simulink model "UoA_1"  (R2014b)
settings: Solver=ode1  StartTime=0.0  StopTime=10000  FixedStep=0.01  RelTol=1e-3
libraries: UoA_3D_LRd_2008 x100
settings Model: SimulationMode=rapid-accelerator  Creator=eyip002-admin  LastModifiedBy=nall426
settings DataIOCC: LimitDataPoints=off  SignalLogging=off  DSMLogging=off  VisualizeSimOutput=off
settings HardwareCC: ProdHWDeviceType=ASIC/FPGA->ASIC/FPGA  TargetBitPerLong=64  TargetBitPerPointer=64  TargetIntDivRoundTo=Zero  TargetEndianess=LittleEndian  TargetWordSize=64  TargetHWDeviceType=Intel->x86-64  ProdEqTarget=off
settings GRTTargetCC: MatFileLogging=off

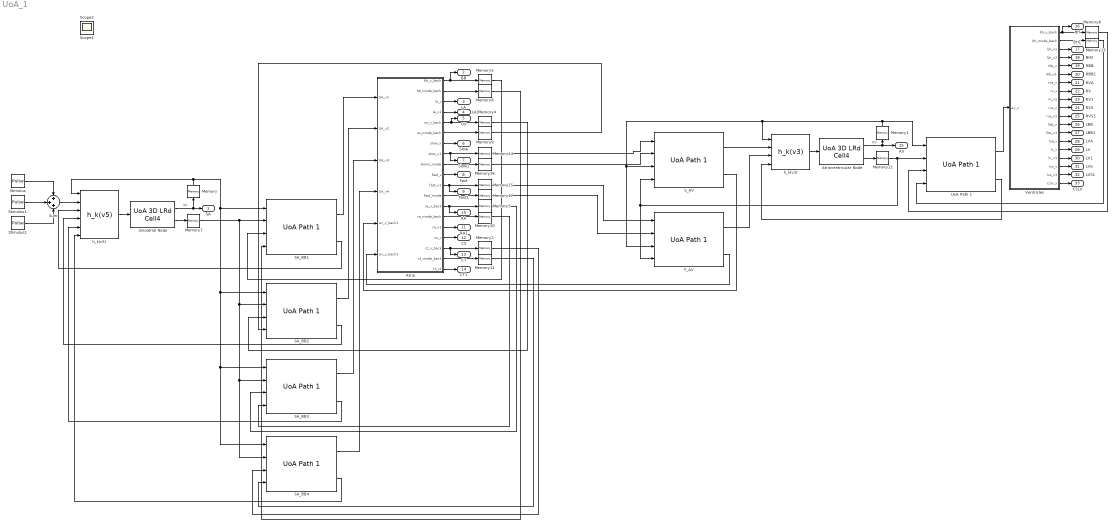
== system UoA_1 ==
  Atria : Subsystem
  Atrioventricular Node : UoA_3D_LRd_2008/UoA 3D LRd Cell4  V_T=44.5  V_R=30  V_O_max=131.1  alpha0_x=-0.0087  alpha1_x=-0.0236  alpha2_x=-0.0069  alpha3_x=-0.0332  alpha0_y=-0.1909  alpha1_y=-0.0455  alpha2_y=0.0759  alpha3_y=0.0200  alpha0_z=-0.1904  alpha1_z=-0.0129  alpha2_z=6.8265  alpha3_z=0.0020  v_n_R_max=0.04  i_st_gx=0.7772  i_st_gy=0.0589  i_st_gz=0.2766
  F_AV : UoA_3D_LRd_2008/UoA Path 1  cell1_conduction_time=10  cell2_conduction_time=10  cell1_charge_time=10  cell2_charge_time=10
  Memory{,1..17} (18 alike) : Memory
  SA_BB{1..4} (4 alike) : UoA_3D_LRd_2008/UoA Path 1  cell1_conduction_time=20  cell2_conduction_time=20  cell1_charge_time=10  cell2_charge_time=10
  S_AV : UoA_3D_LRd_2008/UoA Path 1  cell1_conduction_time=15  cell2_conduction_time=15  cell1_charge_time=10  cell2_charge_time=10
  Sinoatrial Node : UoA_3D_LRd_2008/UoA 3D LRd Cell4  V_T=44.5  V_R=30  V_O_max=131.1  alpha0_x=-0.0087  alpha1_x=-0.0236  alpha2_x=-0.0069  alpha3_x=-0.0332  alpha0_y=-0.1909  alpha1_y=-0.0455  alpha2_y=0.0759  alpha3_y=0.0200  alpha0_z=-0.1904  alpha1_z=-0.0129  alpha2_z=6.8265  alpha3_z=0.0020  v_n_R_max=0.04  i_st_gx=0.7772  i_st_gy=0.0589  i_st_gz=0.2766
  Stimulus : DiscretePulseGenerator  PulseType=Time based  Amplitude=131.1*2  Period=1000  PulseWidth=1.5  PhaseDelay=10
  Stimulus1 : DiscretePulseGenerator  PulseType=Time based  Amplitude=131.1*2  Period=1000  PulseWidth=1.5  PhaseDelay=415
  Stimulus2 : DiscretePulseGenerator  PulseType=Time based  Amplitude=131.1*2  Period=1000  PulseWidth=1.5  PhaseDelay=815
  Sum : Sum  Inputs=+++
  UoA Path 1 : UoA_3D_LRd_2008/UoA Path 1  cell1_conduction_time=30  cell2_conduction_time=30  cell1_charge_time=10  cell2_charge_time=10
  Ventricles : Subsystem
  h_k(v3) : UoA_3D_LRd_2008/h_k(v3)  A_m=10*10  C_m=1/(10*10)  G_1=10*10  G_2=10*10  G_3=10*10  s_1=1/10  s_2=1/10  s_3=1/10  d_1=8  d_2=8  d_3=10
  h_k(v5) : UoA_3D_LRd_2008/h_k(v5)  A_m=10*10  C_m=1/(10*10)  G_1=10*10  G_2=10*10  G_3=10*10  G_4=10*10  G_5=10*10  s_1=1/10  s_2=1/10  s_3=1/10  s_4=1/10  s_5=1/10  d_1=1  d_2=10  d_3=10  d_4=10  d_5=10
  SA : Outport
  BB : Outport  Port=2
  LA : Outport  Port=3
  LA1 : Outport  Port=4
  OS : Outport  Port=5
  Slow : Outport  Port=6
  Slow1 : Outport  Port=7
  Fast : Outport  Port=8
  Fast1 : Outport  Port=9
  RA : Outport  Port=10
  RA1 : Outport  Port=11
  CS : Outport  Port=12
  CT : Outport  Port=13
  CT1 : Outport  Port=14
  AV : Outport  Port=15
  BH : Outport  Port=16
  BH1 : Outport  Port=17
  BH2 : Outport  Port=18
  RBB : Outport  Port=19
  RBB1 : Outport  Port=20
  RVA : Outport  Port=21
  RV : Outport  Port=22
  RV1 : Outport  Port=23
  RVS : Outport  Port=24
  RVS1 : Outport  Port=25
  LBB : Outport  Port=26
  LBB1 : Outport  Port=27
  LVA : Outport  Port=28
  LV : Outport  Port=29
  LV1 : Outport  Port=30
  LVS : Outport  Port=31
  LVS1 : Outport  Port=32
  CSLV : Outport  Port=33
  Scope1 : Scope  NumInputPorts=5
      settings: TimeRange=1000  YMin=-1~-5~-5~-5~-5  YMax=150~150~150~150~150
  Scope2 : Scope  NumInputPorts=12
      settings: TimeRange=1000  YMin=0~-1~-1~-1~-1~-1~-1~-1~-1~-1~-1~-1  YMax=1~1~1~1~1~1~1~1~1~1~1~1  SaveName=ScopeData2
  wires:
  Sinoatrial Node/1 -> SA/1, Memory/1  "SA"
  h_k(v5)/1 -> Sinoatrial Node/1
  Memory/1 -> h_k(v5)/1, SA_BB1/1, SA_BB2/1, SA_BB3/1, SA_BB4/1
  Atrioventricular Node/1 -> AV/1, Memory1/1  "AV"
  Atria/8(slow_v1) -> Slow1/1, Memory14/1
  h_k(v3)/1 -> Atrioventricular Node/1
  Atria/11(fast_v1) -> Fast1/1, Memory15/1
  Ventricles/7(rva_v) -> RVA/1
  Atria/17(ct_v_back) -> CT/1, Memory2/1
  Atria/13(ra_v_back) -> RA/1, Memory3/1
  Atria/5(os_v_back) -> OS/1, Memory4/1
  Atria/1(bb_v_back) -> BB/1, Memory5/1
  Ventricles/1(bh_v_back) -> Memory6/1, BH/1
  Memory2/1 -> SA_BB4/3
  Memory3/1 -> SA_BB3/3
  Memory4/1 -> SA_BB2/3
  Memory5/1 -> SA_BB1/3
  Memory6/1 -> UoA Path 1/3
  Sinoatrial Node/2 -> Memory7/1
  SA_BB1/1 -> Atria/1(SA_v1)
  Atria/2(bb_mode_back) -> Memory8/1
  Memory8/1 -> SA_BB1/4
  SA_BB1/2 -> h_k(v5)/3
  Atria/6(os_mode_back) -> Memory9/1
  Memory9/1 -> SA_BB2/4
  SA_BB2/2 -> h_k(v5)/4
  SA_BB2/1 -> Atria/2(SA_v2)
  Atria/14(ra_mode_back) -> Memory10/1
  Memory10/1 -> SA_BB3/4
  SA_BB3/1 -> Atria/3(SA_v3)
  SA_BB3/2 -> h_k(v5)/5
  Memory7/1 -> SA_BB3/2, SA_BB4/2, SA_BB2/2, SA_BB1/2
  Atria/18(ct_mode_back) -> Memory11/1
  Memory11/1 -> SA_BB4/4
  SA_BB4/1 -> Atria/4(SA_v4)
  SA_BB4/2 -> h_k(v5)/6
  Memory1/1 -> UoA Path 1/1, h_k(v3)/1, F_AV/3, S_AV/3
  Atrioventricular Node/2 -> Memory12/1
  Memory12/1 -> S_AV/4, F_AV/4, UoA Path 1/2
  UoA Path 1/1 -> Ventricles/1(av_v)
  Ventricles/2(bh_mode_back) -> Memory13/1
  Memory13/1 -> UoA Path 1/4
  UoA Path 1/2 -> h_k(v3)/4
  Memory14/1 -> S_AV/1
  Memory15/1 -> F_AV/1
  Atria/9(slow1_mode) -> Memory16/1
  Atria/12(fast_mode) -> Memory17/1
  Memory16/1 -> S_AV/2
  S_AV/1 -> h_k(v3)/2
  S_AV/2 -> Atria/5(av_v_back1)
  Memory17/1 -> F_AV/2
  F_AV/1 -> h_k(v3)/3
  F_AV/2 -> Atria/6(av_v_back2)
  Atria/4(la_v1) -> LA1/1
  Atria/3(la_v) -> LA/1
  Atria/7(slow_v) -> Slow/1
  Atria/10(fast_v) -> Fast/1
  Atria/15(ra_v1) -> RA1/1
  Atria/16(cs_v) -> CS/1
  Atria/19(ct_v1) -> CT1/1
  Ventricles/3(bh_v1) -> BH1/1
  Ventricles/4(bh_v2) -> BH2/1
  Ventricles/5(rbb_v) -> RBB/1
  Ventricles/6(rbb_v1) -> RBB1/1
  Ventricles/8(rv_v) -> RV/1
  Ventricles/9(rv_v1) -> RV1/1
  Ventricles/10(rvs_v) -> RVS/1
  Ventricles/11(rvs_v1) -> RVS1/1
  Ventricles/12(lbb_v) -> LBB/1
  Ventricles/13(lbb_v1) -> LBB1/1
  Ventricles/14(lva_v) -> LVA/1
  Ventricles/15(lv_v) -> LV/1
  Ventricles/16(lv_v1) -> LV1/1
  Ventricles/17(lvs_v) -> LVS/1
  Ventricles/18(lvs_v1) -> LVS1/1
  Ventricles/19(cslv_v) -> CSLV/1
  Sum/1 -> h_k(v5)/2
  Stimulus/1 -> Sum/1
  Stimulus1/1 -> Sum/2
  Stimulus2/1 -> Sum/3

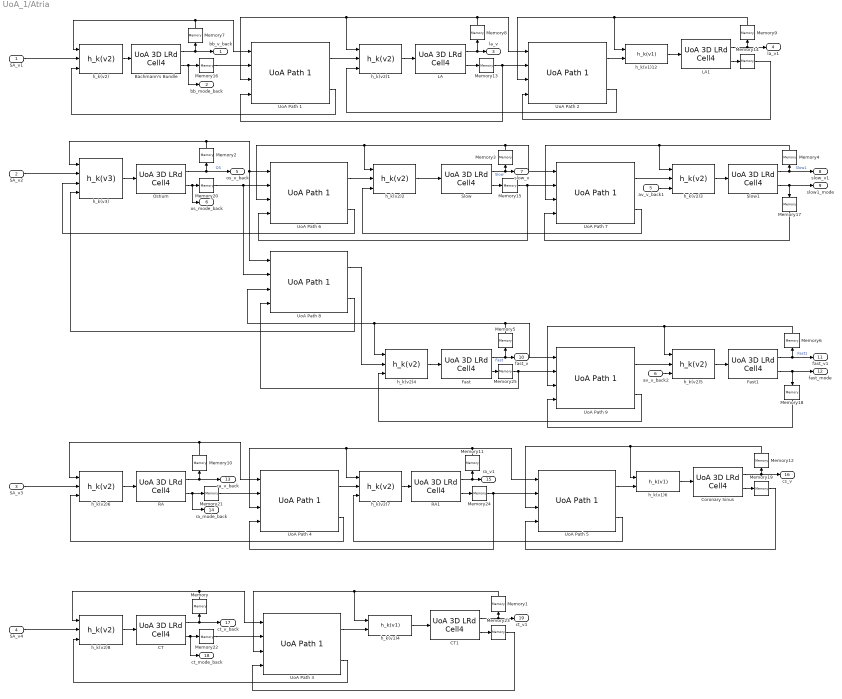
== system UoA_1/Atria ==
  SA_v1 : Inport
  SA_v2 : Inport  Port=2
  SA_v3 : Inport  Port=3
  SA_v4 : Inport  Port=4
  av_v_back1 : Inport  Port=5
  av_v_back2 : Inport  Port=6
  Bachmann's Bundle : UoA_3D_LRd_2008/UoA 3D LRd Cell4  V_T=44.5  V_R=30  V_O_max=131.1  alpha0_x=-0.0087  alpha1_x=-0.0236  alpha2_x=-0.0069  alpha3_x=-0.0332  alpha0_y=-0.1909  alpha1_y=-0.0455  alpha2_y=0.0759  alpha3_y=0.0200  alpha0_z=-0.1904  alpha1_z=-0.0129  alpha2_z=6.8265  alpha3_z=0.0020  v_n_R_max=0.04  i_st_gx=0.7772  i_st_gy=0.0589  i_st_gz=0.2766
  CT : UoA_3D_LRd_2008/UoA 3D LRd Cell4  V_T=44.5  V_R=30  V_O_max=131.1  alpha0_x=-0.0087  alpha1_x=-0.0236  alpha2_x=-0.0069  alpha3_x=-0.0332  alpha0_y=-0.1909  alpha1_y=-0.0455  alpha2_y=0.0759  alpha3_y=0.0200  alpha0_z=-0.1904  alpha1_z=-0.0129  alpha2_z=6.8265  alpha3_z=0.0020  v_n_R_max=0.04  i_st_gx=0.7772  i_st_gy=0.0589  i_st_gz=0.2766
  CT1 : UoA_3D_LRd_2008/UoA 3D LRd Cell4  V_T=44.5  V_R=30  V_O_max=131.1  alpha0_x=-0.0087  alpha1_x=-0.0236  alpha2_x=-0.0069  alpha3_x=-0.0332  alpha0_y=-0.1909  alpha1_y=-0.0455  alpha2_y=0.0759  alpha3_y=0.0200  alpha0_z=-0.1904  alpha1_z=-0.0129  alpha2_z=6.8265  alpha3_z=0.0020  v_n_R_max=0.04  i_st_gx=0.7772  i_st_gy=0.0589  i_st_gz=0.2766
  Coronary Sinus : UoA_3D_LRd_2008/UoA 3D LRd Cell4  V_T=44.5  V_R=30  V_O_max=131.1  alpha0_x=-0.0087  alpha1_x=-0.0236  alpha2_x=-0.0069  alpha3_x=-0.0332  alpha0_y=-0.1909  alpha1_y=-0.0455  alpha2_y=0.0759  alpha3_y=0.0200  alpha0_z=-0.1904  alpha1_z=-0.0129  alpha2_z=6.8265  alpha3_z=0.0020  v_n_R_max=0.04  i_st_gx=0.7772  i_st_gy=0.0589  i_st_gz=0.2766
  Fast : UoA_3D_LRd_2008/UoA 3D LRd Cell4  V_T=44.5  V_R=30  V_O_max=131.1  alpha0_x=-0.0087  alpha1_x=-0.0236  alpha2_x=-0.0069  alpha3_x=-0.0332  alpha0_y=-0.1909  alpha1_y=-0.0455  alpha2_y=0.0759  alpha3_y=0.0180  alpha0_z=-0.1904  alpha1_z=-0.0129  alpha2_z=6.8265  alpha3_z=0.0020  v_n_R_max=0.04  i_st_gx=0.7772  i_st_gy=0.0589  i_st_gz=0.2766
  Fast1 : UoA_3D_LRd_2008/UoA 3D LRd Cell4  V_T=44.5  V_R=30  V_O_max=131.1  alpha0_x=-0.0087  alpha1_x=-0.0236  alpha2_x=-0.0069  alpha3_x=-0.0332  alpha0_y=-0.1909  alpha1_y=-0.0455  alpha2_y=0.0759  alpha3_y=0.0180  alpha0_z=-0.1904  alpha1_z=-0.0129  alpha2_z=6.8265  alpha3_z=0.0020  v_n_R_max=0.04  i_st_gx=0.7772  i_st_gy=0.0589  i_st_gz=0.2766
  LA : UoA_3D_LRd_2008/UoA 3D LRd Cell4  V_T=44.5  V_R=30  V_O_max=131.1  alpha0_x=-0.0087  alpha1_x=-0.0236  alpha2_x=-0.0069  alpha3_x=-0.0332  alpha0_y=-0.1909  alpha1_y=-0.0455  alpha2_y=0.0759  alpha3_y=0.0200  alpha0_z=-0.1904  alpha1_z=-0.0129  alpha2_z=6.8265  alpha3_z=0.0020  v_n_R_max=0.04  i_st_gx=0.7772  i_st_gy=0.0589  i_st_gz=0.2766
  LA1 : UoA_3D_LRd_2008/UoA 3D LRd Cell4  V_T=44.5  V_R=30  V_O_max=131.1  alpha0_x=-0.0087  alpha1_x=-0.0236  alpha2_x=-0.0069  alpha3_x=-0.0332  alpha0_y=-0.1909  alpha1_y=-0.0455  alpha2_y=0.0759  alpha3_y=0.0200  alpha0_z=-0.1904  alpha1_z=-0.0129  alpha2_z=6.8265  alpha3_z=0.0020  v_n_R_max=0.04  i_st_gx=0.7772  i_st_gy=0.0589  i_st_gz=0.2766
  Memory{,1..25} (26 alike) : Memory
  Ostium : UoA_3D_LRd_2008/UoA 3D LRd Cell4  V_T=44.5  V_R=30  V_O_max=131.1  alpha0_x=-0.0087  alpha1_x=-0.0236  alpha2_x=-0.0069  alpha3_x=-0.0332  alpha0_y=-0.1909  alpha1_y=-0.0455  alpha2_y=0.0759  alpha3_y=0.0200  alpha0_z=-0.1904  alpha1_z=-0.0129  alpha2_z=6.8265  alpha3_z=0.0020  v_n_R_max=0.04  i_st_gx=0.7772  i_st_gy=0.0589  i_st_gz=0.2766
  RA : UoA_3D_LRd_2008/UoA 3D LRd Cell4  V_T=44.5  V_R=30  V_O_max=131.1  alpha0_x=-0.0087  alpha1_x=-0.0236  alpha2_x=-0.0069  alpha3_x=-0.0332  alpha0_y=-0.1909  alpha1_y=-0.0455  alpha2_y=0.0759  alpha3_y=0.0200  alpha0_z=-0.1904  alpha1_z=-0.0129  alpha2_z=6.8265  alpha3_z=0.0020  v_n_R_max=0.04  i_st_gx=0.7772  i_st_gy=0.0589  i_st_gz=0.2766
  RA1 : UoA_3D_LRd_2008/UoA 3D LRd Cell4  V_T=44.5  V_R=30  V_O_max=131.1  alpha0_x=-0.0087  alpha1_x=-0.0236  alpha2_x=-0.0069  alpha3_x=-0.0332  alpha0_y=-0.1909  alpha1_y=-0.0455  alpha2_y=0.0759  alpha3_y=0.0200  alpha0_z=-0.1904  alpha1_z=-0.0129  alpha2_z=6.8265  alpha3_z=0.0020  v_n_R_max=0.04  i_st_gx=0.7772  i_st_gy=0.0589  i_st_gz=0.2766
  Slow : UoA_3D_LRd_2008/UoA 3D LRd Cell4  V_T=44.5  V_R=30  V_O_max=131.1  alpha0_x=-0.0087  alpha1_x=-0.0236  alpha2_x=-0.0069  alpha3_x=-0.0332  alpha0_y=-0.1909  alpha1_y=-0.0455  alpha2_y=0.0759  alpha3_y=0.0200  alpha0_z=-0.1904  alpha1_z=-0.0129  alpha2_z=6.8265  alpha3_z=0.0020  v_n_R_max=0.04  i_st_gx=0.7772  i_st_gy=0.0589  i_st_gz=0.2766
  Slow1 : UoA_3D_LRd_2008/UoA 3D LRd Cell4  V_T=44.5  V_R=30  V_O_max=131.1  alpha0_x=-0.0087  alpha1_x=-0.0236  alpha2_x=-0.0069  alpha3_x=-0.0332  alpha0_y=-0.1909  alpha1_y=-0.0455  alpha2_y=0.0759  alpha3_y=0.0200  alpha0_z=-0.1904  alpha1_z=-0.0129  alpha2_z=6.8265  alpha3_z=0.0020  v_n_R_max=0.04  i_st_gx=0.7772  i_st_gy=0.0589  i_st_gz=0.2766
  UoA Path 1 : UoA_3D_LRd_2008/UoA Path 1  cell1_conduction_time=30  cell2_conduction_time=30  cell1_charge_time=10  cell2_charge_time=10
  UoA Path 2 : UoA_3D_LRd_2008/UoA Path 1  cell1_conduction_time=40  cell2_conduction_time=40  cell1_charge_time=10  cell2_charge_time=10
  UoA Path {3..5,8..9} (5 alike) : UoA_3D_LRd_2008/UoA Path 1  cell1_conduction_time=20  cell2_conduction_time=20  cell1_charge_time=10  cell2_charge_time=10
  UoA Path 6 : UoA_3D_LRd_2008/UoA Path 1  cell1_conduction_time=30  cell2_conduction_time=30  cell1_charge_time=10  cell2_charge_time=10
  UoA Path 7 : UoA_3D_LRd_2008/UoA Path 1  cell1_conduction_time=30  cell2_conduction_time=30  cell1_charge_time=10  cell2_charge_time=10
  h_k(v1)12 : UoA_3D_LRd_2008/h_k(v1)  A_m=10*10  C_m=1/(10*10)  G_1=10*10  s_1=1/10  d_1=10
  h_k(v1)4 : UoA_3D_LRd_2008/h_k(v1)  A_m=10*10  C_m=1/(10*10)  G_1=10*10  s_1=1/10  d_1=10
  h_k(v1)6 : UoA_3D_LRd_2008/h_k(v1)  A_m=10*10  C_m=1/(10*10)  G_1=10*10  s_1=1/10  d_1=10
  h_k(v2){,1..8} (9 alike) : UoA_3D_LRd_2008/h_k(v2)  A_m=10*10  C_m=1/(10*10)  G_1=10*10  G_2=10*10  s_1=1/10  s_2=1/10  d_1=10  d_2=10
  h_k(v3) : UoA_3D_LRd_2008/h_k(v3)  A_m=10*10  C_m=1/(10*10)  G_1=10*10  G_2=10*10  G_3=10*10  s_1=1/10  s_2=1/10  s_3=1/10  d_1=1  d_2=10  d_3=10
  bb_v_back : Outport
  bb_mode_back : Outport  Port=2
  la_v : Outport  Port=3
  la_v1 : Outport  Port=4
  os_v_back : Outport  Port=5
  os_mode_back : Outport  Port=6
  slow_v : Outport  Port=7
  slow_v1 : Outport  Port=8
  slow1_mode : Outport  Port=9
  fast_v : Outport  Port=10
  fast_v1 : Outport  Port=11
  fast_mode : Outport  Port=12
  ra_v_back : Outport  Port=13
  ra_mode_back : Outport  Port=14
  ra_v1 : Outport  Port=15
  cs_v : Outport  Port=16
  ct_v_back : Outport  Port=17
  ct_mode_back : Outport  Port=18
  ct_v1 : Outport  Port=19
  wires:
  CT/1 -> Memory/1, ct_v_back/1
  CT1/1 -> ct_v1/1, Memory1/1
  h_k(v2)8/1 -> CT/1
  Memory/1 -> h_k(v2)8/1, UoA Path 3/1
  h_k(v1)4/1 -> CT1/1
  Memory1/1 -> UoA Path 3/3, h_k(v1)4/1
  h_k(v3)/1 -> Ostium/1
  Memory2/1 -> h_k(v3)/1, UoA Path 8/1, UoA Path 6/1
  SA_v1/1 -> h_k(v2)/2
  h_k(v2)2/1 -> Slow/1
  Memory3/1 -> UoA Path 6/3, h_k(v2)2/1, UoA Path 7/1
  h_k(v2)3/1 -> Slow1/1
  Memory4/1 -> h_k(v2)3/1, UoA Path 7/3
  Slow/1 -> slow_v/1, Memory3/1  "Slow"
  h_k(v2)4/1 -> Fast/1
  Ostium/1 -> Memory2/1, os_v_back/1  "OS"
  h_k(v2)5/1 -> Fast1/1
  Memory6/1 -> h_k(v2)5/1, UoA Path 9/3
  Fast/1 -> fast_v/1, Memory5/1  "Fast"
  Slow1/1 -> slow_v1/1, Memory4/1  "Slow1"
  Fast1/1 -> fast_v1/1, Memory6/1  "Fast1"
  h_k(v2)/1 -> Bachmann's Bundle/1
  Memory7/1 -> UoA Path 1/1, h_k(v2)/1
  h_k(v2)1/1 -> LA/1
  Memory8/1 -> UoA Path 2/1, h_k(v2)1/1, UoA Path 1/3
  h_k(v1)12/1 -> LA1/1
  Memory9/1 -> h_k(v1)12/1, UoA Path 2/3
  LA/1 -> la_v/1, Memory8/1
  Bachmann's Bundle/1 -> bb_v_back/1, Memory7/1
  LA1/1 -> la_v1/1, Memory9/1
  h_k(v2)6/1 -> RA/1
  Memory10/1 -> h_k(v2)6/1, UoA Path 4/1
  h_k(v2)7/1 -> RA1/1
  Memory11/1 -> h_k(v2)7/1, UoA Path 4/3, UoA Path 5/1
  h_k(v1)6/1 -> Coronary Sinus/1
  Memory12/1 -> h_k(v1)6/1, UoA Path 5/3
  RA1/1 -> ra_v1/1, Memory11/1
  RA/1 -> ra_v_back/1, Memory10/1
  Coronary Sinus/1 -> cs_v/1, Memory12/1
  av_v_back1/1 -> h_k(v2)3/3
  Memory14/1 -> UoA Path 2/4
  UoA Path 6/2 -> h_k(v3)/3
  Memory5/1 -> h_k(v2)4/1, UoA Path 8/3, UoA Path 9/1
  UoA Path 7/2 -> h_k(v2)2/3
  LA1/2 -> Memory14/1
  CT1/2 -> Memory23/1
  Slow1/2 -> Memory17/1, slow1_mode/1
  Fast1/2 -> Memory18/1, fast_mode/1
  Ostium/2 -> Memory20/1, os_mode_back/1
  SA_v2/1 -> h_k(v3)/2
  SA_v3/1 -> h_k(v2)6/2
  SA_v4/1 -> h_k(v2)8/2
  av_v_back2/1 -> h_k(v2)5/3
  LA/2 -> Memory13/1
  Memory13/1 -> UoA Path 1/4, UoA Path 2/2
  UoA Path 1/1 -> h_k(v2)1/2
  UoA Path 1/2 -> h_k(v2)/3
  UoA Path 2/2 -> h_k(v2)1/3
  UoA Path 2/1 -> h_k(v1)12/2
  Bachmann's Bundle/2 -> Memory16/1, bb_mode_back/1
  UoA Path 3/1 -> h_k(v1)4/2
  CT/2 -> ct_mode_back/1, Memory22/1
  Memory23/1 -> UoA Path 3/4
  UoA Path 3/2 -> h_k(v2)8/3
  RA/2 -> ra_mode_back/1, Memory21/1
  UoA Path 4/1 -> h_k(v2)7/2
  RA1/2 -> Memory24/1
  Memory24/1 -> UoA Path 5/2, UoA Path 4/4
  UoA Path 4/2 -> h_k(v2)6/3
  UoA Path 5/1 -> h_k(v1)6/2
  UoA Path 5/2 -> h_k(v2)7/3
  Coronary Sinus/2 -> Memory19/1
  Memory19/1 -> UoA Path 5/4
  Memory21/1 -> UoA Path 4/2
  Memory22/1 -> UoA Path 3/2
  Memory16/1 -> UoA Path 1/2
  Memory20/1 -> UoA Path 8/2, UoA Path 6/2
  UoA Path 6/1 -> h_k(v2)2/2
  Slow/2 -> Memory15/1
  Memory15/1 -> UoA Path 7/2, UoA Path 6/4
  Memory17/1 -> UoA Path 7/4
  UoA Path 7/1 -> h_k(v2)3/2
  UoA Path 8/1 -> h_k(v2)4/2
  UoA Path 8/2 -> h_k(v3)/4
  Fast/2 -> Memory25/1
  Memory25/1 -> UoA Path 9/2, UoA Path 8/4
  UoA Path 9/2 -> h_k(v2)4/3
  UoA Path 9/1 -> h_k(v2)5/2
  Memory18/1 -> UoA Path 9/4

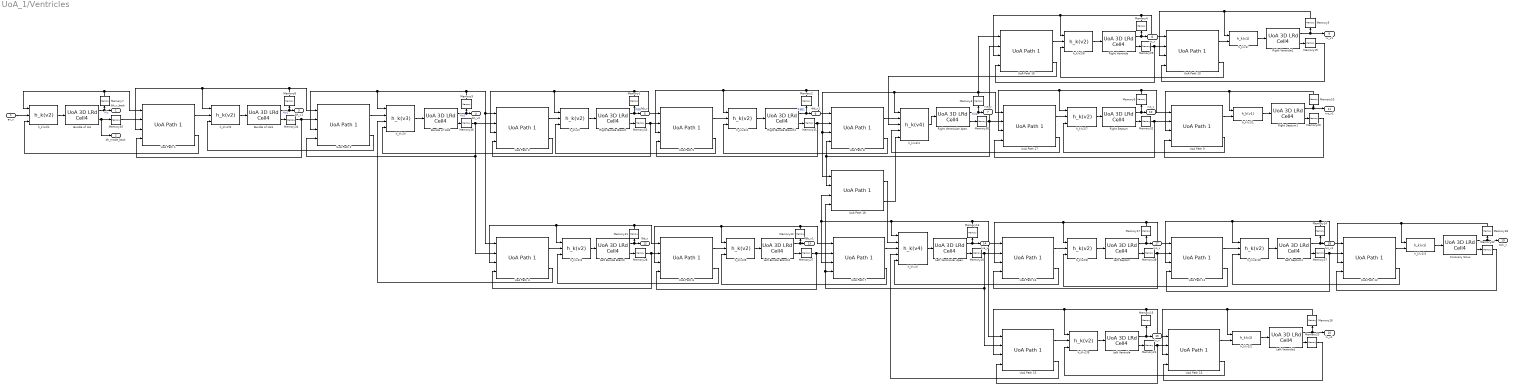
== system UoA_1/Ventricles ==
  av_v : Inport
  Bundle of His : UoA_3D_LRd_2008/UoA 3D LRd Cell4  V_T=44.5  V_R=30  V_O_max=131.1  alpha0_x=-0.0087  alpha1_x=-0.0236  alpha2_x=-0.0069  alpha3_x=-0.0332  alpha0_y=-0.1909  alpha1_y=-0.0455  alpha2_y=0.0759  alpha3_y=0.0110  alpha0_z=-0.1904  alpha1_z=-0.0129  alpha2_z=6.8265  alpha3_z=0.0020  v_n_R_max=0.04  i_st_gx=0.7772  i_st_gy=0.0589  i_st_gz=0.2766
  Bundle of His1 : UoA_3D_LRd_2008/UoA 3D LRd Cell4  V_T=44.5  V_R=30  V_O_max=131.1  alpha0_x=-0.0087  alpha1_x=-0.0236  alpha2_x=-0.0069  alpha3_x=-0.0332  alpha0_y=-0.1909  alpha1_y=-0.0455  alpha2_y=0.0759  alpha3_y=0.0110  alpha0_z=-0.1904  alpha1_z=-0.0129  alpha2_z=6.8265  alpha3_z=0.0020  v_n_R_max=0.04  i_st_gx=0.7772  i_st_gy=0.0589  i_st_gz=0.2766
  Bundle of His2 : UoA_3D_LRd_2008/UoA 3D LRd Cell4  V_T=44.5  V_R=30  V_O_max=131.1  alpha0_x=-0.0087  alpha1_x=-0.0236  alpha2_x=-0.0069  alpha3_x=-0.0332  alpha0_y=-0.1909  alpha1_y=-0.0455  alpha2_y=0.0759  alpha3_y=0.0110  alpha0_z=-0.1904  alpha1_z=-0.0129  alpha2_z=6.8265  alpha3_z=0.0020  v_n_R_max=0.04  i_st_gx=0.7772  i_st_gy=0.0589  i_st_gz=0.2766
  Coronary Sinus : UoA_3D_LRd_2008/UoA 3D LRd Cell4  V_T=44.5  V_R=30  V_O_max=131.1  alpha0_x=-0.0087  alpha1_x=-0.0236  alpha2_x=-0.0069  alpha3_x=-0.0332  alpha0_y=-0.1909  alpha1_y=-0.0455  alpha2_y=0.0759  alpha3_y=0.0110  alpha0_z=-0.1904  alpha1_z=-0.0129  alpha2_z=6.8265  alpha3_z=0.0020  v_n_R_max=0.04  i_st_gx=0.7772  i_st_gy=0.0589  i_st_gz=0.2766
  Left Bundle Branch : UoA_3D_LRd_2008/UoA 3D LRd Cell4  V_T=44.5  V_R=30  V_O_max=131.1  alpha0_x=-0.0087  alpha1_x=-0.0236  alpha2_x=-0.0069  alpha3_x=-0.0332  alpha0_y=-0.1909  alpha1_y=-0.0455  alpha2_y=0.0759  alpha3_y=0.0110  alpha0_z=-0.1904  alpha1_z=-0.0129  alpha2_z=6.8265  alpha3_z=0.0020  v_n_R_max=0.04  i_st_gx=0.7772  i_st_gy=0.0589  i_st_gz=0.2766
  Left Bundle Branch1 : UoA_3D_LRd_2008/UoA 3D LRd Cell4  V_T=44.5  V_R=30  V_O_max=131.1  alpha0_x=-0.0087  alpha1_x=-0.0236  alpha2_x=-0.0069  alpha3_x=-0.0332  alpha0_y=-0.1909  alpha1_y=-0.0455  alpha2_y=0.0759  alpha3_y=0.0110  alpha0_z=-0.1904  alpha1_z=-0.0129  alpha2_z=6.8265  alpha3_z=0.0020  v_n_R_max=0.04  i_st_gx=0.7772  i_st_gy=0.0589  i_st_gz=0.2766
  Left Septum : UoA_3D_LRd_2008/UoA 3D LRd Cell4  V_T=44.5  V_R=30  V_O_max=131.1  alpha0_x=-0.0087  alpha1_x=-0.0236  alpha2_x=-0.0069  alpha3_x=-0.0332  alpha0_y=-0.1909  alpha1_y=-0.0455  alpha2_y=0.0759  alpha3_y=0.0110  alpha0_z=-0.1904  alpha1_z=-0.0129  alpha2_z=6.8265  alpha3_z=0.0020  v_n_R_max=0.04  i_st_gx=0.7772  i_st_gy=0.0589  i_st_gz=0.2766
  Left Septum1 : UoA_3D_LRd_2008/UoA 3D LRd Cell4  V_T=44.5  V_R=30  V_O_max=131.1  alpha0_x=-0.0087  alpha1_x=-0.0236  alpha2_x=-0.0069  alpha3_x=-0.0332  alpha0_y=-0.1909  alpha1_y=-0.0455  alpha2_y=0.0759  alpha3_y=0.0110  alpha0_z=-0.1904  alpha1_z=-0.0129  alpha2_z=6.8265  alpha3_z=0.0020  v_n_R_max=0.04  i_st_gx=0.7772  i_st_gy=0.0589  i_st_gz=0.2766
  Left Ventricle : UoA_3D_LRd_2008/UoA 3D LRd Cell4  V_T=44.5  V_R=30  V_O_max=131.1  alpha0_x=-0.0087  alpha1_x=-0.0236  alpha2_x=-0.0069  alpha3_x=-0.0332  alpha0_y=-0.1909  alpha1_y=-0.0455  alpha2_y=0.0759  alpha3_y=0.0110  alpha0_z=-0.1904  alpha1_z=-0.0129  alpha2_z=6.8265  alpha3_z=0.0020  v_n_R_max=0.04  i_st_gx=0.7772  i_st_gy=0.0589  i_st_gz=0.2766
  Left Ventricle1 : UoA_3D_LRd_2008/UoA 3D LRd Cell4  V_T=44.5  V_R=30  V_O_max=131.1  alpha0_x=-0.0087  alpha1_x=-0.0236  alpha2_x=-0.0069  alpha3_x=-0.0332  alpha0_y=-0.1909  alpha1_y=-0.0455  alpha2_y=0.0759  alpha3_y=0.0110  alpha0_z=-0.1904  alpha1_z=-0.0129  alpha2_z=6.8265  alpha3_z=0.0020  v_n_R_max=0.04  i_st_gx=0.7772  i_st_gy=0.0589  i_st_gz=0.2766
  Left Ventricular Apex : UoA_3D_LRd_2008/UoA 3D LRd Cell4  V_T=44.5  V_R=30  V_O_max=131.1  alpha0_x=-0.0087  alpha1_x=-0.0236  alpha2_x=-0.0069  alpha3_x=-0.0332  alpha0_y=-0.1909  alpha1_y=-0.0455  alpha2_y=0.0759  alpha3_y=0.0110  alpha0_z=-0.1904  alpha1_z=-0.0129  alpha2_z=6.8265  alpha3_z=0.0020  v_n_R_max=0.04  i_st_gx=0.7772  i_st_gy=0.0589  i_st_gz=0.2766
  Memory{1..23,26..38} (36 alike) : Memory
  Right Bundle Branch : UoA_3D_LRd_2008/UoA 3D LRd Cell4  V_T=44.5  V_R=30  V_O_max=131.1  alpha0_x=-0.0087  alpha1_x=-0.0236  alpha2_x=-0.0069  alpha3_x=-0.0332  alpha0_y=-0.1909  alpha1_y=-0.0455  alpha2_y=0.0759  alpha3_y=0.0110  alpha0_z=-0.1904  alpha1_z=-0.0129  alpha2_z=6.8265  alpha3_z=0.0020  v_n_R_max=0.04  i_st_gx=0.7772  i_st_gy=0.0589  i_st_gz=0.2766
  Right Bundle Branch1 : UoA_3D_LRd_2008/UoA 3D LRd Cell4  V_T=44.5  V_R=30  V_O_max=131.1  alpha0_x=-0.0087  alpha1_x=-0.0236  alpha2_x=-0.0069  alpha3_x=-0.0332  alpha0_y=-0.1909  alpha1_y=-0.0455  alpha2_y=0.0759  alpha3_y=0.0110  alpha0_z=-0.1904  alpha1_z=-0.0129  alpha2_z=6.8265  alpha3_z=0.0020  v_n_R_max=0.04  i_st_gx=0.7772  i_st_gy=0.0589  i_st_gz=0.2766
  Right Septum : UoA_3D_LRd_2008/UoA 3D LRd Cell4  V_T=44.5  V_R=30  V_O_max=131.1  alpha0_x=-0.0087  alpha1_x=-0.0236  alpha2_x=-0.0069  alpha3_x=-0.0332  alpha0_y=-0.1909  alpha1_y=-0.0455  alpha2_y=0.0759  alpha3_y=0.0110  alpha0_z=-0.1904  alpha1_z=-0.0129  alpha2_z=6.8265  alpha3_z=0.0020  v_n_R_max=0.04  i_st_gx=0.7772  i_st_gy=0.0589  i_st_gz=0.2766
  Right Septum1 : UoA_3D_LRd_2008/UoA 3D LRd Cell4  V_T=44.5  V_R=30  V_O_max=131.1  alpha0_x=-0.0087  alpha1_x=-0.0236  alpha2_x=-0.0069  alpha3_x=-0.0332  alpha0_y=-0.1909  alpha1_y=-0.0455  alpha2_y=0.0759  alpha3_y=0.0110  alpha0_z=-0.1904  alpha1_z=-0.0129  alpha2_z=6.8265  alpha3_z=0.0020  v_n_R_max=0.04  i_st_gx=0.7772  i_st_gy=0.0589  i_st_gz=0.2766
  Right Ventricle : UoA_3D_LRd_2008/UoA 3D LRd Cell4  V_T=44.5  V_R=30  V_O_max=131.1  alpha0_x=-0.0087  alpha1_x=-0.0236  alpha2_x=-0.0069  alpha3_x=-0.0332  alpha0_y=-0.1909  alpha1_y=-0.0455  alpha2_y=0.0759  alpha3_y=0.0110  alpha0_z=-0.1904  alpha1_z=-0.0129  alpha2_z=6.8265  alpha3_z=0.0020  v_n_R_max=0.04  i_st_gx=0.7772  i_st_gy=0.0589  i_st_gz=0.2766
  Right Ventricle1 : UoA_3D_LRd_2008/UoA 3D LRd Cell4  V_T=44.5  V_R=30  V_O_max=131.1  alpha0_x=-0.0087  alpha1_x=-0.0236  alpha2_x=-0.0069  alpha3_x=-0.0332  alpha0_y=-0.1909  alpha1_y=-0.0455  alpha2_y=0.0759  alpha3_y=0.0110  alpha0_z=-0.1904  alpha1_z=-0.0129  alpha2_z=6.8265  alpha3_z=0.0020  v_n_R_max=0.04  i_st_gx=0.7772  i_st_gy=0.0589  i_st_gz=0.2766
  Right Ventricular Apex : UoA_3D_LRd_2008/UoA 3D LRd Cell4  V_T=44.5  V_R=30  V_O_max=131.1  alpha0_x=-0.0087  alpha1_x=-0.0236  alpha2_x=-0.0069  alpha3_x=-0.0332  alpha0_y=-0.1909  alpha1_y=-0.0455  alpha2_y=0.0759  alpha3_y=0.0110  alpha0_z=-0.1904  alpha1_z=-0.0129  alpha2_z=6.8265  alpha3_z=0.0020  v_n_R_max=0.04  i_st_gx=0.7772  i_st_gy=0.0589  i_st_gz=0.2766
  UoA Path {1..4,9..10,12,15} (8 alike) : UoA_3D_LRd_2008/UoA Path 1  cell1_conduction_time=20  cell2_conduction_time=20  cell1_charge_time=10  cell2_charge_time=10
  UoA Path 11 : UoA_3D_LRd_2008/UoA Path 1  cell1_conduction_time=15  cell2_conduction_time=15  cell1_charge_time=10  cell2_charge_time=10
  UoA Path 13 : UoA_3D_LRd_2008/UoA Path 1  cell1_conduction_time=30  cell2_conduction_time=30  cell1_charge_time=10  cell2_charge_time=10
  UoA Path 14 : UoA_3D_LRd_2008/UoA Path 1  cell1_conduction_time=15  cell2_conduction_time=15  cell1_charge_time=10  cell2_charge_time=10
  UoA Path 16 : UoA_3D_LRd_2008/UoA Path 1  cell1_conduction_time=10  cell2_conduction_time=10  cell1_charge_time=10  cell2_charge_time=10
  UoA Path 17 : UoA_3D_LRd_2008/UoA Path 1  cell1_conduction_time=15  cell2_conduction_time=15  cell1_charge_time=10  cell2_charge_time=10
  UoA Path {5..8,18} (5 alike) : UoA_3D_LRd_2008/UoA Path 1  cell1_conduction_time=5  cell2_conduction_time=5  cell1_charge_time=10  cell2_charge_time=10
  h_k(v1){,1..3} (4 alike) : UoA_3D_LRd_2008/h_k(v1)  A_m=10*10  C_m=1/(10*10)  G_1=10*10  s_1=1/10  d_1=10
  h_k(v2){,1..10} (11 alike) : UoA_3D_LRd_2008/h_k(v2)  A_m=10*10  C_m=1/(10*10)  G_1=10*10  G_2=10*10  s_1=1/10  s_2=1/10  d_1=10  d_2=10
  h_k(v3) : UoA_3D_LRd_2008/h_k(v3)  A_m=10*10  C_m=1/(10*10)  G_1=10*10  G_2=10*10  G_3=10*10  s_1=1/10  s_2=1/10  s_3=1/10  d_1=1  d_2=10  d_3=10
  h_k(v4) : UoA_3D_LRd_2008/h_k(v4)  A_m=10*10  C_m=1/(10*10)  G_1=10*10  G_2=10*10  G_3=10*10  G_4=10*10  s_1=1/10  s_2=1/10  s_3=1/10  s_4=1/10  d_1=1  d_2=10  d_3=10  d_4=10
  h_k(v4)1 : UoA_3D_LRd_2008/h_k(v4)  A_m=10*10  C_m=1/(10*10)  G_1=10*10  G_2=10*10  G_3=10*10  G_4=10*10  s_1=1/10  s_2=1/10  s_3=1/10  s_4=1/10  d_1=1  d_2=10  d_3=10  d_4=10
  bh_v_back : Outport
  bh_mode_back : Outport  Port=2
  bh_v1 : Outport  Port=3
  bh_v2 : Outport  Port=4
  rbb_v : Outport  Port=5
  rbb_v1 : Outport  Port=6
  rva_v : Outport  Port=7
  rv_v : Outport  Port=8
  rv_v1 : Outport  Port=9
  rvs_v : Outport  Port=10
  rvs_v1 : Outport  Port=11
  lbb_v : Outport  Port=12
  lbb_v1 : Outport  Port=13
  lva_v : Outport  Port=14
  lv_v : Outport  Port=15
  lv_v1 : Outport  Port=16
  lvs_v : Outport  Port=17
  lvs_v1 : Outport  Port=18
  cslv_v : Outport  Port=19
  wires:
  av_v/1 -> h_k(v2)1/2
  h_k(v2)1/1 -> Bundle of His/1
  Memory7/1 -> UoA Path 1/1, h_k(v2)1/1
  h_k(v2)2/1 -> Bundle of His1/1
  Memory8/1 -> UoA Path 2/1, UoA Path 1/3, h_k(v2)2/1
  h_k(v3)/1 -> Bundle of His2/1
  Memory9/1 -> h_k(v3)/1, UoA Path 2/3, UoA Path 4/1, UoA Path 3/1
  Bundle of His1/1 -> bh_v1/1, Memory8/1  "His1"
  Bundle of His/1 -> Memory7/1, bh_v_back/1  "His"
  h_k(v2)/1 -> Right Bundle Branch/1
  Memory1/1 -> UoA Path 5/1, h_k(v2)/1, UoA Path 3/3
  h_k(v2)4/1 -> Right Bundle Branch1/1
  Memory2/1 -> h_k(v2)4/1, UoA Path 5/3, UoA Path 8/1
  h_k(v4)1/1 -> Right Ventricular Apex/1
  Memory3/1 -> h_k(v4)1/1, UoA Path 8/3, UoA Path 18/1, UoA Path 17/1, UoA Path 16/1
  Right Bundle Branch1/1 -> rbb_v1/1, Memory2/1  "RBB1"
  Right Bundle Branch/1 -> rbb_v/1, Memory1/1  "RBB"
  h_k(v2)6/1 -> Right Ventricle/1
  Memory4/1 -> UoA Path 10/1, h_k(v2)6/1, UoA Path 16/3
  h_k(v1)/1 -> Right Ventricle1/1
  Right Ventricle/1 -> rv_v/1, Memory4/1
  Right Ventricle1/1 -> rv_v1/1, Memory5/1
  h_k(v2)7/1 -> Right Septum/1
  h_k(v1)1/1 -> Right Septum1/1
  Memory10/1 -> h_k(v1)1/1, UoA Path 9/3
  Right Septum/1 -> rvs_v/1, Memory6/1
  Bundle of His2/1 -> bh_v2/1, Memory9/1  "His2"
  h_k(v2)3/1 -> Left Bundle Branch/1
  Memory11/1 -> UoA Path 6/1, UoA Path 4/3, h_k(v2)3/1
  h_k(v2)5/1 -> Left Bundle Branch1/1
  h_k(v4)/1 -> Left Ventricular Apex/1
  Left Bundle Branch1/1 -> lbb_v1/1, Memory12/1
  Memory13/1 -> UoA Path 15/1, UoA Path 14/1, h_k(v4)/1, UoA Path 7/3, UoA Path 18/3
  Left Bundle Branch/1 -> lbb_v/1, Memory11/1
  h_k(v2)9/1 -> Left Ventricle/1
  h_k(v1)2/1 -> Left Ventricle1/1
  Memory16/1 -> h_k(v1)2/1, UoA Path 13/3
  Left Ventricle/1 -> lv_v/1, Memory15/1
  Left Ventricular Apex/1 -> lva_v/1, Memory13/1
  Left Ventricle1/1 -> lv_v1/1, Memory16/1
  h_k(v2)8/1 -> Left Septum/1
  h_k(v2)10/1 -> Left Septum1/1
  Memory14/1 -> UoA Path 12/1, h_k(v2)10/1, UoA Path 11/3
  Left Septum/1 -> lvs_v/1, Memory17/1
  Left Septum1/1 -> lvs_v1/1, Memory14/1
  h_k(v1)3/1 -> Coronary Sinus/1
  Memory18/1 -> h_k(v1)3/1, UoA Path 12/3
  Coronary Sinus/1 -> cslv_v/1, Memory18/1
  Right Ventricular Apex/1 -> rva_v/1, Memory3/1  "RVA"
  Right Septum1/1 -> rvs_v1/1, Memory10/1
  UoA Path 9/2 -> h_k(v2)7/3
  Memory15/1 -> UoA Path 13/1, h_k(v2)9/1, UoA Path 15/3
  UoA Path 14/2 -> h_k(v4)/5
  UoA Path 4/2 -> h_k(v3)/3
  Memory6/1 -> UoA Path 9/1, UoA Path 17/3, h_k(v2)7/1
  UoA Path 3/2 -> h_k(v3)/4
  UoA Path 1/2 -> h_k(v2)1/3
  Right Ventricle1/2 -> Memory19/1
  Right Septum1/2 -> Memory20/1
  Coronary Sinus/2 -> Memory22/1
  Right Ventricular Apex/2 -> Memory30/1
  Bundle of His/2 -> bh_mode_back/1, Memory35/1
  Memory35/1 -> UoA Path 1/2
  UoA Path 1/1 -> h_k(v2)2/2
  Bundle of His1/2 -> Memory34/1
  Memory34/1 -> UoA Path 2/2, UoA Path 1/4
  UoA Path 2/2 -> h_k(v2)2/3
  UoA Path 2/1 -> h_k(v3)/2
  Bundle of His2/2 -> Memory36/1
  Memory36/1 -> UoA Path 3/2, UoA Path 4/2, UoA Path 2/4
  UoA Path 3/1 -> h_k(v2)/2
  Right Bundle Branch/2 -> Memory33/1
  Memory33/1 -> UoA Path 5/2, UoA Path 3/4
  UoA Path 5/2 -> h_k(v2)/3
  UoA Path 5/1 -> h_k(v2)4/2
  Right Bundle Branch1/2 -> Memory31/1
  Memory31/1 -> UoA Path 8/2, UoA Path 5/4
  UoA Path 4/1 -> h_k(v2)3/2
  Left Bundle Branch/2 -> Memory28/1
  Memory28/1 -> UoA Path 6/2, UoA Path 4/4
  UoA Path 6/2 -> h_k(v2)3/3
  UoA Path 6/1 -> h_k(v2)5/2
  Memory12/1 -> UoA Path 7/1, UoA Path 6/3, h_k(v2)5/1
  Left Bundle Branch1/2 -> Memory27/1
  Memory27/1 -> UoA Path 7/2, UoA Path 6/4
  UoA Path 8/2 -> h_k(v2)4/3
  Memory30/1 -> UoA Path 16/2, UoA Path 17/2, UoA Path 8/4, UoA Path 18/2
  UoA Path 7/2 -> h_k(v2)5/3
  UoA Path 7/1 -> h_k(v4)/3
  Left Ventricular Apex/2 -> Memory26/1
  Memory26/1 -> UoA Path 14/2, UoA Path 15/2, UoA Path 18/4, UoA Path 7/4
  Right Septum/2 -> Memory32/1
  Memory32/1 -> UoA Path 17/4, UoA Path 9/2
  UoA Path 8/1 -> h_k(v4)1/2
  UoA Path 9/1 -> h_k(v1)1/2
  Memory20/1 -> UoA Path 9/4
  Right Ventricle/2 -> Memory29/1
  Memory29/1 -> UoA Path 16/4, UoA Path 10/2
  UoA Path 10/1 -> h_k(v1)/2
  UoA Path 10/2 -> h_k(v2)6/3
  Memory19/1 -> UoA Path 10/4
  Memory5/1 -> UoA Path 10/3, h_k(v1)/1
  Left Ventricle1/2 -> Memory23/1
  Left Septum1/2 -> Memory37/1
  Left Septum/2 -> Memory38/1
  Memory17/1 -> UoA Path 14/3, h_k(v2)8/1, UoA Path 11/1
  UoA Path 11/1 -> h_k(v2)10/2
  Memory37/1 -> UoA Path 12/2, UoA Path 11/4
  UoA Path 11/2 -> h_k(v2)8/3
  UoA Path 12/1 -> h_k(v1)3/2
  UoA Path 12/2 -> h_k(v2)10/3
  Memory22/1 -> UoA Path 12/4
  Left Ventricle/2 -> Memory21/1
  UoA Path 13/1 -> h_k(v1)2/2
  Memory23/1 -> UoA Path 13/4
  UoA Path 13/2 -> h_k(v2)9/3
  Memory21/1 -> UoA Path 15/4, UoA Path 13/2
  Memory38/1 -> UoA Path 14/4, UoA Path 11/2
  UoA Path 14/1 -> h_k(v2)8/2
  UoA Path 15/1 -> h_k(v2)9/2
  UoA Path 15/2 -> h_k(v4)/4
  UoA Path 16/1 -> h_k(v2)6/2
  UoA Path 16/2 -> h_k(v4)1/3
  UoA Path 17/1 -> h_k(v2)7/2
  UoA Path 17/2 -> h_k(v4)1/4
  UoA Path 18/1 -> h_k(v4)/2
  UoA Path 18/2 -> h_k(v4)1/5
